simulink model "TheveninSimulink"  (R2016a)
settings: Solver=VariableStepAuto  StartTime=0.0  StopTime=10.0  RelTol=1e-3
undefined symbols (not defined in the file): C1, eta, Q, R0, R1
libraries: simulink x2
settings Model: Creator=Matej  LastModifiedBy=Matej

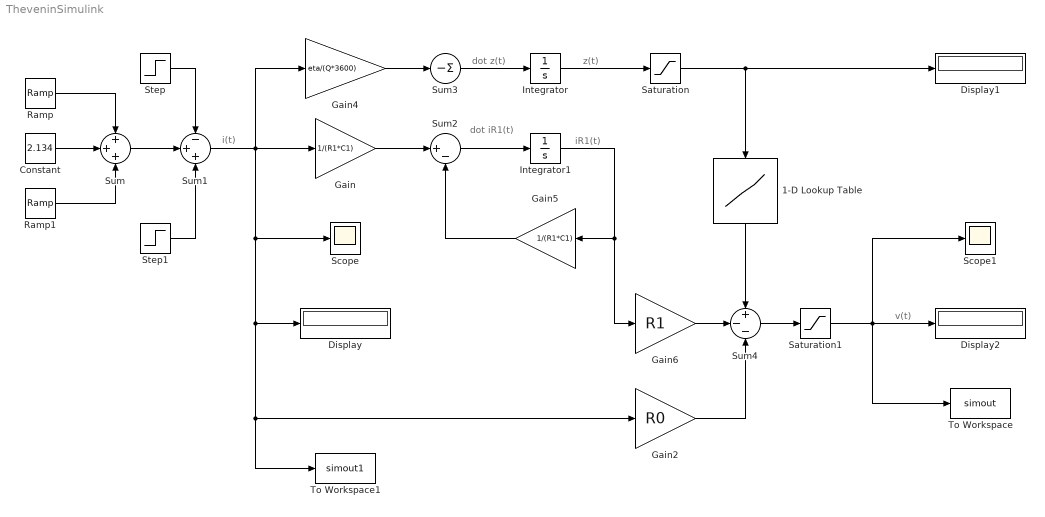
== system TheveninSimulink ==
  note: v(t)
  note: z(t)
  note: iR1(t)
  note: dot iR1(t)
  note: dot z(t)
  note: i(t)
  1-D Lookup Table : Lookup_n-D  NumberOfTableDimensions=1  BreakpointsForDimension1=[-5:5]  Table=tanh([-5:5])  InternalRulePriority=Speed  RndMeth=Simplest  InputSameDT=on
  Constant : Constant  Value=2.134
  Display : Display
  Display1 : Display
  Display2 : Display
  Gain : Gain  Gain=1/(R1*C1)
  Gain2 : Gain  Gain=R0
  Gain4 : Gain  Gain=eta/(Q*3600)
  Gain5 : Gain  Gain=1/(R1*C1)
  Gain6 : Gain  Gain=R1
  Integrator : Integrator
  Integrator1 : Integrator
  Ramp : simulink/Sources/Ramp  slope=1  start=0  X0=0
  Ramp1 : simulink/Sources/Ramp  slope=1  start=0  X0=0
  Saturation : Saturate
  Saturation1 : Saturate
  Scope : Scope
  Scope1 : Scope
  Step : Step  Before=1  After=0  SampleTime=0
  Step1 : Step  SampleTime=0
  Sum : Sum  Inputs=+++
  Sum1 : Sum  Inputs=-++
  Sum2 : Sum  Inputs=|+-
  Sum3 : Sum  Inputs=-
  Sum4 : Sum  Inputs=+--
  To Workspace : ToWorkspace  VariableName=simout  SaveFormat=Timeseries  SampleTime=-1
  To Workspace1 : ToWorkspace  VariableName=simout1  SaveFormat=Timeseries  SampleTime=-1
  wires:
  Ramp/1 -> Sum/1
  Constant/1 -> Sum/2
  Ramp1/1 -> Sum/3
  Sum/1 -> Sum1/2
  Step/1 -> Sum1/1
  Step1/1 -> Sum1/3
  Gain/1 -> Sum2/1
  Gain4/1 -> Sum3/1
  Sum3/1 -> Integrator/1
  Sum2/1 -> Integrator1/1
  Integrator/1 -> Saturation/1
  Integrator1/1 -> Gain6/1, Gain5/1
  Gain5/1 -> Sum2/2
  Gain6/1 -> Sum4/2
  Gain2/1 -> Sum4/3
  Sum1/1 -> Gain4/1, Scope/1, Display/1, To Workspace1/1, Gain2/1, Gain/1
  1-D Lookup Table/1 -> Sum4/1
  Saturation/1 -> Display1/1, 1-D Lookup Table/1
  Sum4/1 -> Saturation1/1
  Saturation1/1 -> To Workspace/1, Scope1/1, Display2/1
